simulink model "ArregloSeisPorSeis"
settings: Solver=ode23t  StartTime=0.0  StopTime=0.003  RelTol=1e-9  AbsTol=1e-9
values from neighbouring files (symbols this model uses):
  a11 = 300    [matlab1.mat]
  a12 = 200    [matlab1.mat]
  a13 = 100    [matlab1.mat]
  a14 = 100    [matlab1.mat]
  a15 = 100    [matlab1.mat]
  a16 = 100    [matlab1.mat]
  a21 = 200    [matlab1.mat]
  a22 = 100    [matlab1.mat]
  a23 = 100    [matlab1.mat]
  a24 = 1000    [matlab1.mat]
  a25 = 100    [matlab1.mat]
  a26 = 100    [matlab1.mat]
  a31 = 100    [matlab1.mat]
  a32 = 100    [matlab1.mat]
  a33 = 100    [matlab1.mat]
  a34 = 100    [matlab1.mat]
  a35 = 100    [matlab1.mat]
  a36 = 100    [matlab1.mat]
  a41 = 100    [matlab1.mat]
  a42 = 100    [matlab1.mat]
  a43 = 100    [matlab1.mat]
  a44 = 100    [matlab1.mat]
  a45 = 100    [matlab1.mat]
  a46 = 100    [matlab1.mat]
  a51 = 100    [matlab1.mat]
  a52 = 100    [matlab1.mat]
  a53 = 100    [matlab1.mat]
  a54 = 100    [matlab1.mat]
  a55 = 100    [matlab1.mat]
  a56 = 100    [matlab1.mat]
  a61 = 100    [matlab1.mat]
  a62 = 100    [matlab1.mat]
  a63 = 100    [matlab1.mat]
  a64 = 100    [matlab1.mat]
  a65 = 100    [matlab1.mat]
  a66 = 100    [matlab1.mat]
libraries: powerlib x154
(part 1 of 2)
settings Model: Creator=XUAN TRUONG  LastModifiedBy=David
settings SolverCC: AlgebraicLoopSolver=LineSearch  SolverResetMethod=Robust
settings DataIOCC: LimitDataPoints=on  SaveFormat=Array  SignalLoggingSaveFormat=ModelDataLogs  ReturnWorkspaceOutputs=off
settings OptimizationCC: ExpressionDepthLimit=2147483647  LifeSpan=inf  SimCompilerOptimization=Off
settings DebuggingCC: UnderspecifiedInitializationDetection=Classic  MergeDetectMultiDrivingBlocksExec=none  SolverPrmCheckMsg=warning  MultiTaskDSMMsg=warning  MultiTaskCondExecSysMsg=none  FcnCallInpInsideContextMsg=Enable All  StateNameClashWarn=warning  StrictBusMsg=None  SFUnexpectedBacktrackingDiag=warning  SFNoUnconditionalDefaultTransitionDiag=warning
settings HardwareCC: ProdBitPerPointer=32  ProdLargestAtomicFloat=None  ProdIntDivRoundTo=Undefined  ProdEndianess=Unspecified  ProdWordSize=32  ProdHWDeviceType=32-bit Generic
settings ModelReferenceCC: PropagateSignalLabelsOutOfModel=off
settings SFSimCC: SimUseLocalCustomCode=off
settings RTWCC: RTWUseLocalCustomCode=off  IncludeERTFirstTime=on  RTWCompilerOptimization=Off
settings GRTTargetCC: CodeReplacementLibrary=C89/C90 (ANSI)  GeneratePreprocessorConditionals=Disable all  CombineOutputUpdateFcns=off  CPPClassGenCompliant=off  GRTInterface=on

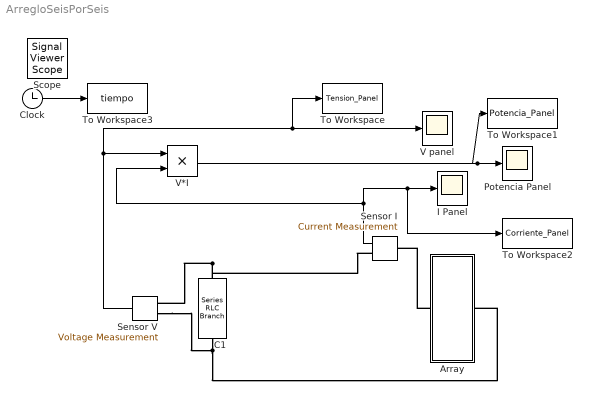
== system ArregloSeisPorSeis ==
  " C1" : powerlib/Elements/Series RLC Branch  LConnTagsString=__new0  RConnTagsString=__new0  BranchType=C  Resistance=5  Inductance=0.05  SetiL0=off  InitialCurrent=0  Capacitance=50e-6  Setx0=on  InitialVoltage=0  Measurements=Branch voltage and current
  Array : Subsystem
  Clock : Clock
  I Panel : Scope
      settings: YMin=0.00012  YMax=0.000137  SaveName=Ip  MaxDataPoints=150000
  Potencia Panel : Scope
      settings: TimeRange=0.003  YMin=0.01  YMax=0.0135  SaveName=P  MaxDataPoints=150000
  Sensor I : powerlib/Measurements/Current Measurement  PhasorSimulation=off  OutputType=Complex  PSBequivalent=0
  Sensor V : powerlib/Measurements/Voltage Measurement  PhasorSimulation=off  OutputType=Complex  PSBequivalent=0
  To Workspace : ToWorkspace  VariableName=Tension_Panel  SampleTime=-1
  To Workspace1 : ToWorkspace  VariableName=Potencia_Panel  SampleTime=-1
  To Workspace2 : ToWorkspace  VariableName=Corriente_Panel  SampleTime=-1
  To Workspace3 : ToWorkspace  VariableName=tiempo  SampleTime=-1
  V panel : Scope
      settings: YMin=130.2  YMax=130.9  SaveName=Vp  MaxDataPoints=150000
  V*I : Product  RndMeth=Zero
  Scope : SignalViewerScope  IOType=viewer  RefreshTime=0.035000
  wires:
  Sensor V/1 -> V*I/1, V panel/1, To Workspace/1
  Sensor I/1 -> V*I/2, I Panel/1, To Workspace2/1
  V*I/1 -> Potencia Panel/1, To Workspace1/1
  Clock/1 -> To Workspace3/1
  connections:
  " C1"/RConn1 -- Sensor V/LConn2 -- Array/RConn1
  " C1"/LConn1 -- Sensor I/RConn1 -- Sensor V/LConn1
  Array/LConn1 -- Sensor I/LConn1

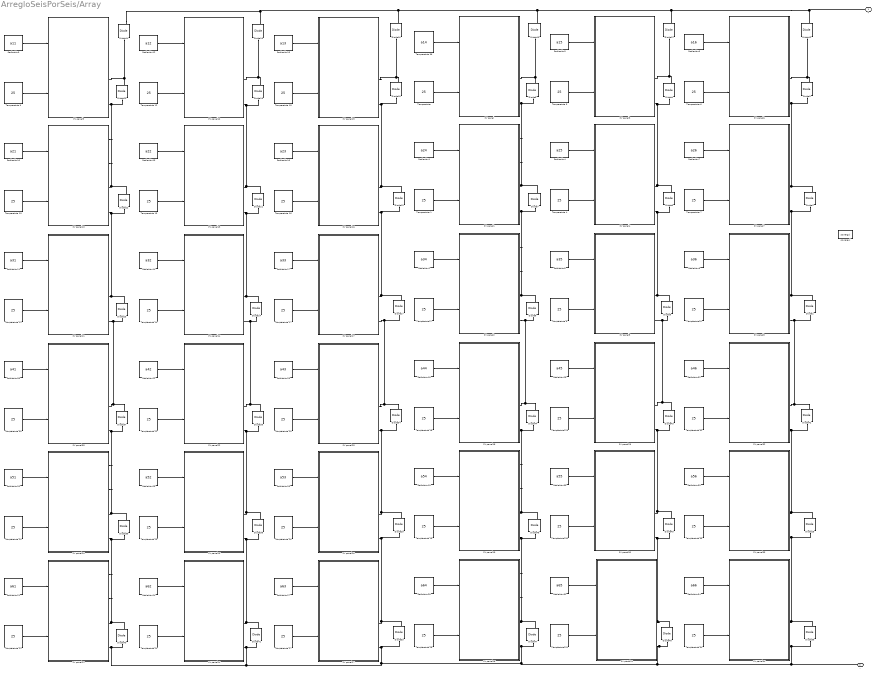
== system ArregloSeisPorSeis/Array ==
  Diode{1..25,29,33..48} (42 alike) : powerlib/Power Electronics/Diode  Ron=0.00001  Lon=0  Vf=0.3  IC=0  UseSnubber=off  Rs=1e10  Cs=1e-9  Measurements=on
  PV panel : Subsystem
      mask Display: image('C:\Users\Mauro\Dropbox\Fuente\Panel (2).jpg')
  PV panel1 : Subsystem
      mask Display: image('C:\Users\Mauro\Dropbox\Fuente\Panel (2).jpg')
  PV panel10 : Subsystem
      mask Display: image('C:\Users\Mauro\Dropbox\Fuente\Panel (2).jpg')
  PV panel11 : Subsystem
      mask Display: image('C:\Users\Mauro\Dropbox\Fuente\Panel (2).jpg')
  PV panel12 : Subsystem
      mask Display: image('C:\Users\Mauro\Dropbox\Fuente\Panel (2).jpg')
  PV panel13 : Subsystem
      mask Display: image('C:\Users\Mauro\Dropbox\Fuente\Panel (2).jpg')
  PV panel14 : Subsystem
      mask Display: image('C:\Users\Mauro\Dropbox\Fuente\Panel (2).jpg')
  PV panel15 : Subsystem
      mask Display: image('C:\Users\Mauro\Dropbox\Fuente\Panel (2).jpg')
  PV panel16 : Subsystem
      mask Display: image('C:\Users\Mauro\Dropbox\Fuente\Panel (2).jpg')
  PV panel17 : Subsystem
      mask Display: image('C:\Users\Mauro\Dropbox\Fuente\Panel (2).jpg')
  PV panel18 : Subsystem
      mask Display: image('C:\Users\Mauro\Dropbox\Fuente\Panel (2).jpg')
  PV panel19 : Subsystem
      mask Display: image('C:\Users\Mauro\Dropbox\Fuente\Panel (2).jpg')
  PV panel2 : Subsystem
      mask Display: image('C:\Users\Mauro\Dropbox\Fuente\Panel (2).jpg')
  PV panel20 : Subsystem
      mask Display: image('C:\Users\Mauro\Dropbox\Fuente\Panel (2).jpg')
  PV panel21 : Subsystem
      mask Display: image('C:\Users\Mauro\Dropbox\Fuente\Panel (2).jpg')
  PV panel22 : Subsystem
      mask Display: image('C:\Users\Mauro\Dropbox\Fuente\Panel (2).jpg')
  PV panel23 : Subsystem
      mask Display: image('C:\Users\Mauro\Dropbox\Fuente\Panel (2).jpg')
  PV panel24 : Subsystem
      mask Display: image('C:\Users\Mauro\Dropbox\Fuente\Panel (2).jpg')
  PV panel25 : Subsystem
      mask Display: image('C:\Users\Mauro\Dropbox\Fuente\Panel (2).jpg')
  PV panel26 : Subsystem
      mask Display: image('C:\Users\Mauro\Dropbox\Fuente\Panel (2).jpg')
  PV panel27 : Subsystem
      mask Display: image('C:\Users\Mauro\Dropbox\Fuente\Panel (2).jpg')
  PV panel28 : Subsystem
      mask Display: image('C:\Users\Mauro\Dropbox\Fuente\Panel (2).jpg')
  PV panel29 : Subsystem
      mask Display: image('C:\Users\Mauro\Dropbox\Fuente\Panel (2).jpg')
  PV panel3 : Subsystem
      mask Display: image('C:\Users\Mauro\Dropbox\Fuente\Panel (2).jpg')
  PV panel30 : Subsystem
      mask Display: image('C:\Users\Mauro\Dropbox\Fuente\Panel (2).jpg')
  PV panel31 : Subsystem
      mask Display: image('C:\Users\Mauro\Dropbox\Fuente\Panel (2).jpg')
  PV panel32 : Subsystem
      mask Display: image('C:\Users\Mauro\Dropbox\Fuente\Panel (2).jpg')
  PV panel33 : Subsystem
      mask Display: image('C:\Users\Mauro\Dropbox\Fuente\Panel (2).jpg')
  PV panel34 : Subsystem
      mask Display: image('C:\Users\Mauro\Dropbox\Fuente\Panel (2).jpg')
  PV panel35 : Subsystem
      mask Display: image('C:\Users\Mauro\Dropbox\Fuente\Panel (2).jpg')
  PV panel4 : Subsystem
      mask Display: image('C:\Users\Mauro\Dropbox\Fuente\Panel (2).jpg')
  PV panel5 : Subsystem
      mask Display: image('C:\Users\Mauro\Dropbox\Fuente\Panel (2).jpg')
  PV panel6 : Subsystem
      mask Display: image('C:\Users\Mauro\Dropbox\Fuente\Panel (2).jpg')
  PV panel7 : Subsystem
      mask Display: image('C:\Users\Mauro\Dropbox\Fuente\Panel (2).jpg')
  PV panel8 : Subsystem
      mask Display: image('C:\Users\Mauro\Dropbox\Fuente\Panel (2).jpg')
  PV panel9 : Subsystem
      mask Display: image('C:\Users\Mauro\Dropbox\Fuente\Panel (2).jpg')
  Radiación1 : Constant  Value=a24
      mask Display: image('C:\Users\Mauro\Dropbox\Fuente\Sol.jpg')
  Radiación10 : Constant  Value=a21
      mask Display: image('C:\Users\Mauro\Dropbox\Fuente\Sol.jpg')
  Radiación11 : Constant  Value=a31
      mask Display: image('C:\Users\Mauro\Dropbox\Fuente\Sol.jpg')
  Radiación12 : Constant  Value=a12
      mask Display: image('C:\Users\Mauro\Dropbox\Fuente\Sol.jpg')
  Radiación13 : Constant  Value=a22
      mask Display: image('C:\Users\Mauro\Dropbox\Fuente\Sol.jpg')
  Radiación14 : Constant  Value=a32
      mask Display: image('C:\Users\Mauro\Dropbox\Fuente\Sol.jpg')
  Radiación15 : Constant  Value=a13
      mask Display: image('C:\Users\Mauro\Dropbox\Fuente\Sol.jpg')
  Radiación16 : Constant  Value=a23
      mask Display: image('C:\Users\Mauro\Dropbox\Fuente\Sol.jpg')
  Radiación17 : Constant  Value=a33
      mask Display: image('C:\Users\Mauro\Dropbox\Fuente\Sol.jpg')
  Radiación18 : Constant  Value=a44
      mask Display: image('C:\Users\Mauro\Dropbox\Fuente\Sol.jpg')
  Radiación19 : Constant  Value=a54
      mask Display: image('C:\Users\Mauro\Dropbox\Fuente\Sol.jpg')
  Radiación2 : Constant  Value=a34
      mask Display: image('C:\Users\Mauro\Dropbox\Fuente\Sol.jpg')
  Radiación20 : Constant  Value=a51
      mask Display: image('C:\Users\Mauro\Dropbox\Fuente\Sol.jpg')
  Radiación21 : Constant  Value=a61
      mask Display: image('C:\Users\Mauro\Dropbox\Fuente\Sol.jpg')
  Radiación22 : Constant  Value=a42
      mask Display: image('C:\Users\Mauro\Dropbox\Fuente\Sol.jpg')
  Radiación23 : Constant  Value=a52
      mask Display: image('C:\Users\Mauro\Dropbox\Fuente\Sol.jpg')
  Radiación24 : Constant  Value=a62
      mask Display: image('C:\Users\Mauro\Dropbox\Fuente\Sol.jpg')
  Radiación25 : Constant  Value=a43
      mask Display: image('C:\Users\Mauro\Dropbox\Fuente\Sol.jpg')
  Radiación26 : Constant  Value=a53
      mask Display: image('C:\Users\Mauro\Dropbox\Fuente\Sol.jpg')
  Radiación27 : Constant  Value=a63
      mask Display: image('C:\Users\Mauro\Dropbox\Fuente\Sol.jpg')
  Radiación28 : Constant  Value=a64
      mask Display: image('C:\Users\Mauro\Dropbox\Fuente\Sol.jpg')
  Radiación29 : Constant  Value=a45
      mask Display: image('C:\Users\Mauro\Dropbox\Fuente\Sol.jpg')
  Radiación3 : Constant  Value=a15
      mask Display: image('C:\Users\Mauro\Dropbox\Fuente\Sol.jpg')
  Radiación30 : Constant  Value=a55
      mask Display: image('C:\Users\Mauro\Dropbox\Fuente\Sol.jpg')
  Radiación31 : Constant  Value=a65
      mask Display: image('C:\Users\Mauro\Dropbox\Fuente\Sol.jpg')
  Radiación32 : Constant  Value=a46
      mask Display: image('C:\Users\Mauro\Dropbox\Fuente\Sol.jpg')
  Radiación33 : Constant  Value=a56
      mask Display: image('C:\Users\Mauro\Dropbox\Fuente\Sol.jpg')
  Radiación34 : Constant  Value=a66
      mask Display: image('C:\Users\Mauro\Dropbox\Fuente\Sol.jpg')
  Radiación35 : Constant  Value=a41
      mask Display: image('C:\Users\Mauro\Dropbox\Fuente\Sol.jpg')
  Radiación4 : Constant  Value=a25
      mask Display: image('C:\Users\Mauro\Dropbox\Fuente\Sol.jpg')
  Radiación5 : Constant  Value=a35
      mask Display: image('C:\Users\Mauro\Dropbox\Fuente\Sol.jpg')
  Radiación6 : Constant  Value=a16
      mask Display: image('C:\Users\Mauro\Dropbox\Fuente\Sol.jpg')
  Radiación7 : Constant  Value=a26
      mask Display: image('C:\Users\Mauro\Dropbox\Fuente\Sol.jpg')
  Radiación8 : Constant  Value=a36
      mask Display: image('C:\Users\Mauro\Dropbox\Fuente\Sol.jpg')
  Radiación9 : Constant  Value=a11
      mask Display: image('C:\Users\Mauro\Dropbox\Fuente\Sol.jpg')
  Temperatuta {,1..35} (36 alike) : Constant  Value=25
      mask Display: image('C:\Users\Mauro\Dropbox\Fuente\Termometro.jpg')
  Temperatuta 36 : Constant  Value=a14
      mask Display: image('C:\Users\Mauro\Dropbox\Fuente\Termometro.jpg')
  powergui : powerlib/powergui  Priority=1  SimulationMode=Discrete  SolverType=Tustin  SampleTime=5e-6  frequency=60  SPID=off  DisableSnubberDevices=off  DisableRonSwitches=off  DisableVfSwitches=off  SwTol=0  Interpol=off  DisplayEquations=off  FunctionMessages=off  frequencyindice=0  Pbase=100e6  ErrMax=1e-4  Iterations=50  UnitsV=kV  UnitsW=MW  echomessages=off  HookPort=off  EnableUseOfTLC=off  x0status=blocks  RestoreLinks=warning  ResistiveCurrentMeasurement=off  Frange=[0:2:500]  Ylog=off  Xlog=on  ShowGrid=off  save=off  variable=ZData  ZoomFFT=off  StartTime=0.0  cycles=1  DisplayStyle=1  fundamental=60  FreqAxis=off  MaxFrequency=1000  frequencyindicesteady=1  RmsSteady=1  display=off  Ts=0  methode=off
  + : PMIOPort  Tag=PMCPort  Port=1  Side=Left
  - : PMIOPort  Tag=PMCPort  Port=2  Side=Right
  wires:
  Radiación2/1 -> PV panel2/1(Radiación)
  Temperatuta 2/1 -> PV panel2/2(Temperatura)
  Radiación3/1 -> PV panel3/1(Radiación)
  Temperatuta 3/1 -> PV panel3/2(Temperatura)
  Radiación4/1 -> PV panel4/1(Radiación)
  Temperatuta 4/1 -> PV panel4/2(Temperatura)
  Radiación5/1 -> PV panel5/1(Radiación)
  Temperatuta 5/1 -> PV panel5/2(Temperatura)
  PV panel1/1(Ipv) -> ?
  PV panel1/2(Vpv) -> ?
  Radiación6/1 -> PV panel6/1(Radiación)
  Temperatuta 6/1 -> PV panel6/2(Temperatura)
  Radiación7/1 -> PV panel7/1(Radiación)
  Temperatuta 7/1 -> PV panel7/2(Temperatura)
  Radiación8/1 -> PV panel8/1(Radiación)
  Temperatuta 8/1 -> PV panel8/2(Temperatura)
  Temperatuta 36/1 -> PV panel/1(Radiación)
  "Temperatuta "/1 -> PV panel/2(Temperatura)
  Radiación1/1 -> PV panel1/1(Radiación)
  Temperatuta 1/1 -> PV panel1/2(Temperatura)
  PV panel2/2(Vpv) -> ?
  PV panel2/1(Ipv) -> ?
  Radiación11/1 -> PV panel11/1(Radiación)
  Temperatuta 11/1 -> PV panel11/2(Temperatura)
  Radiación12/1 -> PV panel12/1(Radiación)
  Temperatuta 12/1 -> PV panel12/2(Temperatura)
  Radiación13/1 -> PV panel13/1(Radiación)
  Temperatuta 13/1 -> PV panel13/2(Temperatura)
  Radiación14/1 -> PV panel14/1(Radiación)
  Temperatuta 14/1 -> PV panel14/2(Temperatura)
  PV panel10/1(Ipv) -> ?
  PV panel10/2(Vpv) -> ?
  Radiación15/1 -> PV panel15/1(Radiación)
  Temperatuta 15/1 -> PV panel15/2(Temperatura)
  Radiación16/1 -> PV panel16/1(Radiación)
  Temperatuta 16/1 -> PV panel16/2(Temperatura)
  Radiación17/1 -> PV panel17/1(Radiación)
  Temperatuta 17/1 -> PV panel17/2(Temperatura)
  Radiación9/1 -> PV panel9/1(Radiación)
  Temperatuta 9/1 -> PV panel9/2(Temperatura)
  Radiación10/1 -> PV panel10/1(Radiación)
  Temperatuta 10/1 -> PV panel10/2(Temperatura)
  Radiación28/1 -> PV panel28/1(Radiación)
  Temperatuta 28/1 -> PV panel28/2(Temperatura)
  Radiación29/1 -> PV panel29/1(Radiación)
  Temperatuta 29/1 -> PV panel29/2(Temperatura)
  Radiación30/1 -> PV panel30/1(Radiación)
  Temperatuta 30/1 -> PV panel30/2(Temperatura)
  Radiación31/1 -> PV panel31/1(Radiación)
  Temperatuta 31/1 -> PV panel31/2(Temperatura)
  PV panel19/1(Ipv) -> ?
  PV panel19/2(Vpv) -> ?
  Radiación32/1 -> PV panel32/1(Radiación)
  Temperatuta 32/1 -> PV panel32/2(Temperatura)
  Radiación33/1 -> PV panel33/1(Radiación)
  Temperatuta 33/1 -> PV panel33/2(Temperatura)
  Radiación34/1 -> PV panel34/1(Radiación)
  Temperatuta 34/1 -> PV panel34/2(Temperatura)
  Radiación18/1 -> PV panel18/1(Radiación)
  Temperatuta 18/1 -> PV panel18/2(Temperatura)
  Radiación19/1 -> PV panel19/1(Radiación)
  Temperatuta 19/1 -> PV panel19/2(Temperatura)
  PV panel28/2(Vpv) -> ?
  PV panel28/1(Ipv) -> ?
  Radiación21/1 -> PV panel21/1(Radiación)
  Temperatuta 21/1 -> PV panel21/2(Temperatura)
  Radiación22/1 -> PV panel22/1(Radiación)
  Temperatuta 22/1 -> PV panel22/2(Temperatura)
  Radiación23/1 -> PV panel23/1(Radiación)
  Temperatuta 23/1 -> PV panel23/2(Temperatura)
  Radiación24/1 -> PV panel24/1(Radiación)
  Temperatuta 24/1 -> PV panel24/2(Temperatura)
  PV panel20/1(Ipv) -> ?
  PV panel20/2(Vpv) -> ?
  Radiación25/1 -> PV panel25/1(Radiación)
  Temperatuta 25/1 -> PV panel25/2(Temperatura)
  Radiación26/1 -> PV panel26/1(Radiación)
  Temperatuta 26/1 -> PV panel26/2(Temperatura)
  Radiación27/1 -> PV panel27/1(Radiación)
  Temperatuta 27/1 -> PV panel27/2(Temperatura)
  Radiación35/1 -> PV panel35/1(Radiación)
  Temperatuta 35/1 -> PV panel35/2(Temperatura)
  Radiación20/1 -> PV panel20/1(Radiación)
  Temperatuta 20/1 -> PV panel20/2(Temperatura)
  PV panel21/2(Vpv) -> ?
  PV panel21/1(Ipv) -> ?
  connections:
  PV panel/RConn2 -- Diode5/LConn1 -- Diode7/RConn1 -- PV panel1/RConn1
  PV panel4/RConn1 -- Diode6/RConn1 -- Diode4/LConn1 -- PV panel3/RConn2
  PV panel7/RConn1 -- Diode1/RConn1 -- Diode3/LConn1 -- PV panel6/RConn2
  PV panel5/RConn1 -- Diode9/RConn1 -- Diode6/LConn1 -- PV panel4/RConn2
  Diode14/RConn1 -- Diode10/RConn1 -- +/RConn1 -- Diode12/RConn1 -- Diode11/RConn1 -- Diode16/RConn1 -- Diode15/RConn1
  PV panel2/RConn1 -- Diode8/RConn1 -- Diode7/LConn1 -- PV panel1/RConn2
  PV panel8/RConn1 -- Diode2/RConn1 -- Diode1/LConn1 -- PV panel7/RConn2
  PV panel18/RConn1 -- Diode44/RConn1 -- Diode8/LConn1 -- PV panel2/RConn2
  PV panel/RConn1 -- Diode5/RConn1 -- Diode10/LConn1
  Diode4/RConn1 -- Diode11/LConn1 -- PV panel3/RConn1
  PV panel6/RConn1 -- Diode3/RConn1 -- Diode12/LConn1
  PV panel9/RConn2 -- Diode20/LConn1 -- Diode22/RConn1 -- PV panel10/RConn1
  PV panel12/RConn2 -- Diode21/RConn1 -- PV panel13/RConn1 -- Diode19/LConn1
  PV panel16/RConn1 -- Diode13/RConn1 -- Diode18/LConn1 -- PV panel15/RConn2
  PV panel13/RConn2 -- Diode24/RConn1 -- PV panel14/RConn1 -- Diode21/LConn1
  PV panel10/RConn2 -- Diode23/RConn1 -- PV panel11/RConn1 -- Diode22/LConn1
  PV panel16/RConn2 -- Diode13/LConn1 -- Diode17/RConn1 -- PV panel17/RConn1
  PV panel9/RConn1 -- Diode20/RConn1 -- Diode14/LConn1
  Diode19/RConn1 -- Diode15/LConn1 -- PV panel12/RConn1
  PV panel15/RConn1 -- Diode18/RConn1 -- Diode16/LConn1
  PV panel18/RConn2 -- Diode44/LConn1 -- Diode46/RConn1 -- PV panel19/RConn1
  PV panel29/RConn2 -- Diode45/RConn1 -- PV panel30/RConn1 -- Diode43/LConn1
  PV panel33/RConn1 -- Diode25/RConn1 -- Diode42/LConn1 -- PV panel32/RConn2
  PV panel30/RConn2 -- Diode48/RConn1 -- PV panel31/RConn1 -- Diode45/LConn1
  PV panel19/RConn2 -- Diode47/RConn1 -- PV panel28/RConn1 -- Diode46/LConn1
  PV panel33/RConn2 -- Diode36/RConn1 -- PV panel34/RConn1 -- Diode25/LConn1
  PV panel27/RConn2 -- Diode33/LConn1 -- Diode36/LConn1 -- PV panel34/RConn2 -- -/RConn1 -- Diode48/LConn1 -- PV panel31/RConn2 -- Diode47/LConn1 -- PV panel28/RConn2 -- Diode40/LConn1 -- PV panel21/RConn2 -- Diode41/LConn1 -- PV panel24/RConn2
  PV panel35/RConn2 -- Diode37/LConn1 -- Diode39/RConn1 -- PV panel20/RConn1
  PV panel22/RConn2 -- Diode35/LConn1 -- Diode38/RConn1 -- PV panel23/RConn1
  PV panel26/RConn1 -- Diode29/RConn1 -- Diode34/LConn1 -- PV panel25/RConn2
  PV panel23/RConn2 -- Diode38/LConn1 -- Diode41/RConn1 -- PV panel24/RConn1
  PV panel20/RConn2 -- Diode39/LConn1 -- Diode40/RConn1 -- PV panel21/RConn1
  PV panel26/RConn2 -- Diode29/LConn1 -- Diode33/RConn1 -- PV panel27/RConn1
  PV panel32/RConn1 -- Diode42/RConn1 -- Diode2/LConn1 -- PV panel8/RConn2
  Diode43/RConn1 -- PV panel5/RConn2 -- Diode9/LConn1 -- PV panel29/RConn1
  Diode35/RConn1 -- PV panel14/RConn2 -- Diode24/LConn1 -- PV panel22/RConn1
  PV panel25/RConn1 -- Diode34/RConn1 -- Diode17/LConn1 -- PV panel17/RConn2
  PV panel35/RConn1 -- Diode23/LConn1 -- PV panel11/RConn2 -- Diode37/RConn1

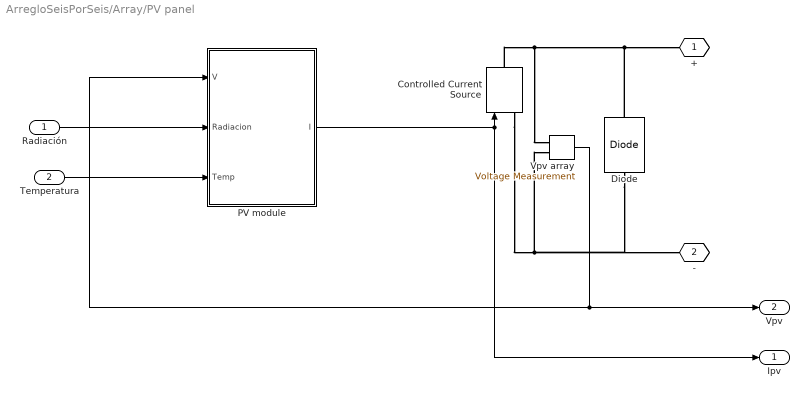
== system ArregloSeisPorSeis/Array/PV panel ==
  Radiación : Inport
  Temperatura : Inport  Port=2
  Controlled Current Source : powerlib/Electrical Sources/Controlled Current Source  Initialize=on  Source_Type=AC  Amplitude=0  Phase=0  Frequency=0  Measurements=None
  Diode : powerlib/Power Electronics/Diode  Ron=0.001  Lon=0  Vf=0  IC=0  UseSnubber=off  Rs=500  Cs=250e-9  Measurements=off
  PV module : MATLAB Function  TreatAsAtomicUnit=on
  Vpv array : powerlib/Measurements/Voltage Measurement  PhasorSimulation=off  OutputType=Complex  PSBequivalent=0
  + : PMIOPort  Tag=PMCPort  Port=1  Side=Right
  - : PMIOPort  Tag=PMCPort  Port=2  Side=Right
  Ipv : Outport
  Vpv : Outport  Port=2
  wires:
  Radiación/1 -> PV module/2(Radiacion)
  Temperatura/1 -> PV module/3(Temp)
  PV module/1(I) -> Controlled Current Source/1, Ipv/1
  Vpv array/1 -> PV module/1(V), Vpv/1
  connections:
  Controlled Current Source/LConn1 -- Diode/LConn1 -- -/RConn1 -- Vpv array/LConn2
  Controlled Current Source/RConn1 -- Diode/RConn1 -- +/RConn1 -- Vpv array/LConn1

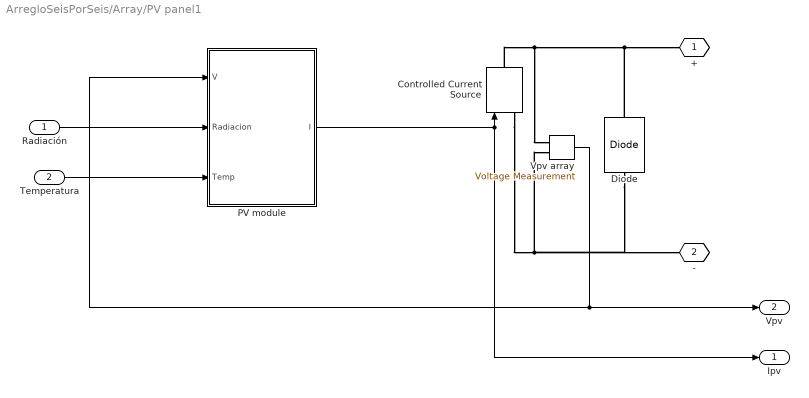
== system ArregloSeisPorSeis/Array/PV panel1 ==
  Radiación : Inport
  Temperatura : Inport  Port=2
  Controlled Current Source : powerlib/Electrical Sources/Controlled Current Source  Initialize=on  Source_Type=AC  Amplitude=0  Phase=0  Frequency=0  Measurements=None
  Diode : powerlib/Power Electronics/Diode  Ron=0.001  Lon=0  Vf=0  IC=0  UseSnubber=off  Rs=500  Cs=250e-9  Measurements=off
  PV module : MATLAB Function  TreatAsAtomicUnit=on
  Vpv array : powerlib/Measurements/Voltage Measurement  PhasorSimulation=off  OutputType=Complex  PSBequivalent=0
  + : PMIOPort  Tag=PMCPort  Port=1  Side=Right
  - : PMIOPort  Tag=PMCPort  Port=2  Side=Right
  Ipv : Outport
  Vpv : Outport  Port=2
  wires:
  Radiación/1 -> PV module/2(Radiacion)
  Temperatura/1 -> PV module/3(Temp)
  PV module/1(I) -> Controlled Current Source/1, Ipv/1
  Vpv array/1 -> PV module/1(V), Vpv/1
  connections:
  Controlled Current Source/LConn1 -- Diode/LConn1 -- -/RConn1 -- Vpv array/LConn2
  Controlled Current Source/RConn1 -- Diode/RConn1 -- +/RConn1 -- Vpv array/LConn1

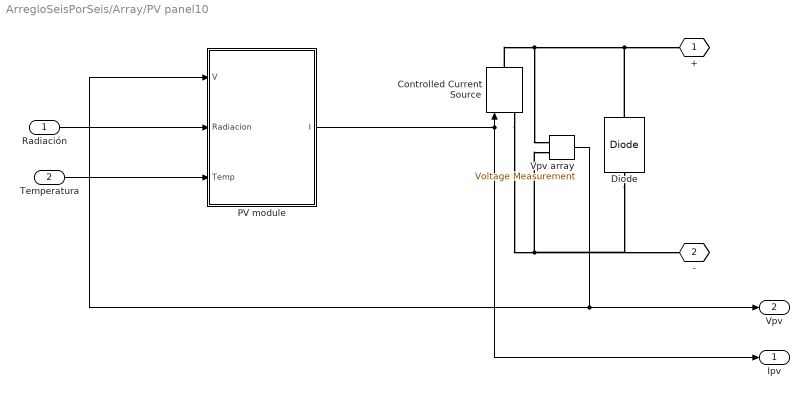
== system ArregloSeisPorSeis/Array/PV panel10 ==
  Radiación : Inport
  Temperatura : Inport  Port=2
  Controlled Current Source : powerlib/Electrical Sources/Controlled Current Source  Initialize=on  Source_Type=AC  Amplitude=0  Phase=0  Frequency=0  Measurements=None
  Diode : powerlib/Power Electronics/Diode  Ron=0.001  Lon=0  Vf=0  IC=0  UseSnubber=off  Rs=500  Cs=250e-9  Measurements=off
  PV module : MATLAB Function  TreatAsAtomicUnit=on
  Vpv array : powerlib/Measurements/Voltage Measurement  PhasorSimulation=off  OutputType=Complex  PSBequivalent=0
  + : PMIOPort  Tag=PMCPort  Port=1  Side=Right
  - : PMIOPort  Tag=PMCPort  Port=2  Side=Right
  Ipv : Outport
  Vpv : Outport  Port=2
  wires:
  Radiación/1 -> PV module/2(Radiacion)
  Temperatura/1 -> PV module/3(Temp)
  PV module/1(I) -> Controlled Current Source/1, Ipv/1
  Vpv array/1 -> PV module/1(V), Vpv/1
  connections:
  Controlled Current Source/LConn1 -- Diode/LConn1 -- -/RConn1 -- Vpv array/LConn2
  Controlled Current Source/RConn1 -- Diode/RConn1 -- +/RConn1 -- Vpv array/LConn1

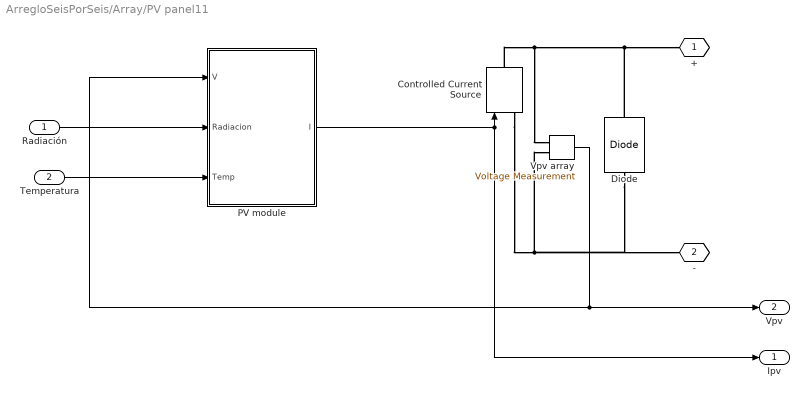
== system ArregloSeisPorSeis/Array/PV panel11 ==
  Radiación : Inport
  Temperatura : Inport  Port=2
  Controlled Current Source : powerlib/Electrical Sources/Controlled Current Source  Initialize=on  Source_Type=AC  Amplitude=0  Phase=0  Frequency=0  Measurements=None
  Diode : powerlib/Power Electronics/Diode  Ron=0.001  Lon=0  Vf=0  IC=0  UseSnubber=off  Rs=500  Cs=250e-9  Measurements=off
  PV module : MATLAB Function  TreatAsAtomicUnit=on
  Vpv array : powerlib/Measurements/Voltage Measurement  PhasorSimulation=off  OutputType=Complex  PSBequivalent=0
  + : PMIOPort  Tag=PMCPort  Port=1  Side=Right
  - : PMIOPort  Tag=PMCPort  Port=2  Side=Right
  Ipv : Outport
  Vpv : Outport  Port=2
  wires:
  Radiación/1 -> PV module/2(Radiacion)
  Temperatura/1 -> PV module/3(Temp)
  PV module/1(I) -> Controlled Current Source/1, Ipv/1
  Vpv array/1 -> PV module/1(V), Vpv/1
  connections:
  Controlled Current Source/LConn1 -- Diode/LConn1 -- -/RConn1 -- Vpv array/LConn2
  Controlled Current Source/RConn1 -- Diode/RConn1 -- +/RConn1 -- Vpv array/LConn1

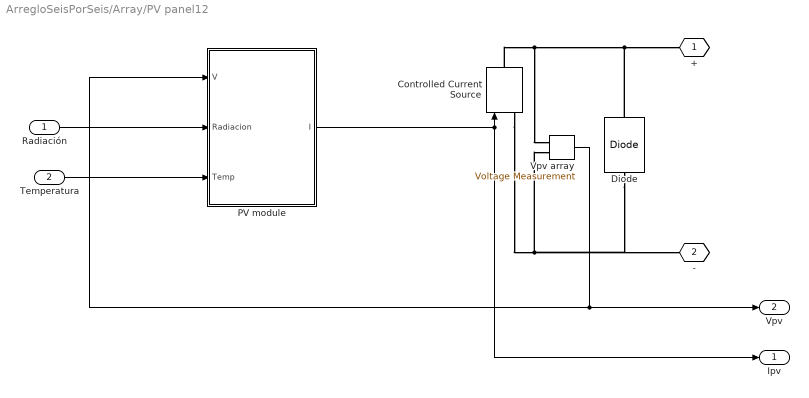
== system ArregloSeisPorSeis/Array/PV panel12 ==
  Radiación : Inport
  Temperatura : Inport  Port=2
  Controlled Current Source : powerlib/Electrical Sources/Controlled Current Source  Initialize=on  Source_Type=AC  Amplitude=0  Phase=0  Frequency=0  Measurements=None
  Diode : powerlib/Power Electronics/Diode  Ron=0.001  Lon=0  Vf=0  IC=0  UseSnubber=off  Rs=500  Cs=250e-9  Measurements=off
  PV module : MATLAB Function  TreatAsAtomicUnit=on
  Vpv array : powerlib/Measurements/Voltage Measurement  PhasorSimulation=off  OutputType=Complex  PSBequivalent=0
  + : PMIOPort  Tag=PMCPort  Port=1  Side=Right
  - : PMIOPort  Tag=PMCPort  Port=2  Side=Right
  Ipv : Outport
  Vpv : Outport  Port=2
  wires:
  Radiación/1 -> PV module/2(Radiacion)
  Temperatura/1 -> PV module/3(Temp)
  PV module/1(I) -> Controlled Current Source/1, Ipv/1
  Vpv array/1 -> PV module/1(V), Vpv/1
  connections:
  Controlled Current Source/LConn1 -- Diode/LConn1 -- -/RConn1 -- Vpv array/LConn2
  Controlled Current Source/RConn1 -- Diode/RConn1 -- +/RConn1 -- Vpv array/LConn1

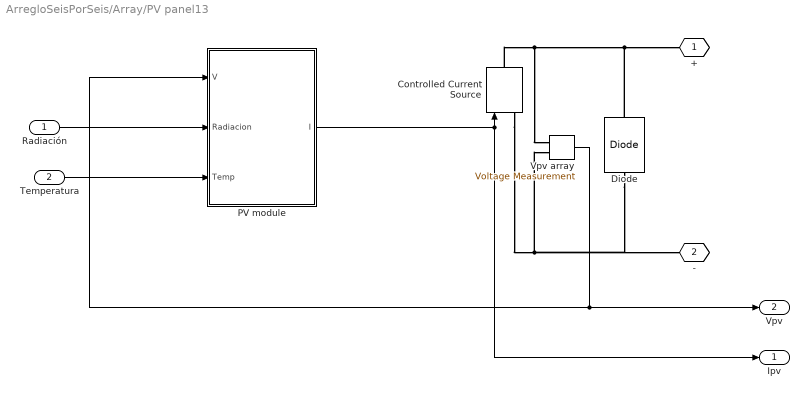
== system ArregloSeisPorSeis/Array/PV panel13 ==
  Radiación : Inport
  Temperatura : Inport  Port=2
  Controlled Current Source : powerlib/Electrical Sources/Controlled Current Source  Initialize=on  Source_Type=AC  Amplitude=0  Phase=0  Frequency=0  Measurements=None
  Diode : powerlib/Power Electronics/Diode  Ron=0.001  Lon=0  Vf=0  IC=0  UseSnubber=off  Rs=500  Cs=250e-9  Measurements=off
  PV module : MATLAB Function  TreatAsAtomicUnit=on
  Vpv array : powerlib/Measurements/Voltage Measurement  PhasorSimulation=off  OutputType=Complex  PSBequivalent=0
  + : PMIOPort  Tag=PMCPort  Port=1  Side=Right
  - : PMIOPort  Tag=PMCPort  Port=2  Side=Right
  Ipv : Outport
  Vpv : Outport  Port=2
  wires:
  Radiación/1 -> PV module/2(Radiacion)
  Temperatura/1 -> PV module/3(Temp)
  PV module/1(I) -> Controlled Current Source/1, Ipv/1
  Vpv array/1 -> PV module/1(V), Vpv/1
  connections:
  Controlled Current Source/LConn1 -- Diode/LConn1 -- -/RConn1 -- Vpv array/LConn2
  Controlled Current Source/RConn1 -- Diode/RConn1 -- +/RConn1 -- Vpv array/LConn1

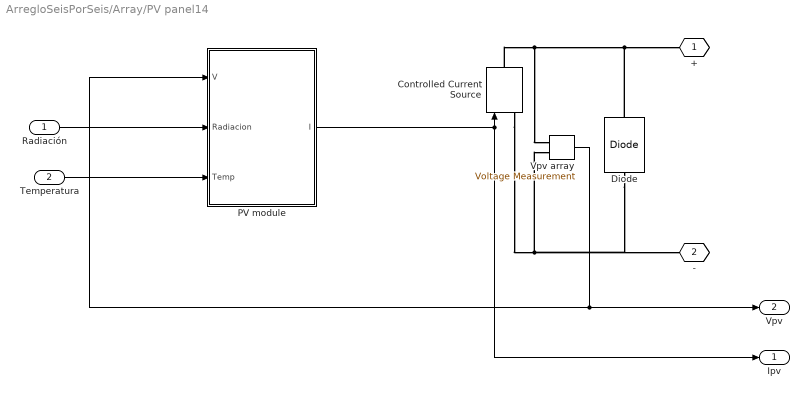
== system ArregloSeisPorSeis/Array/PV panel14 ==
  Radiación : Inport
  Temperatura : Inport  Port=2
  Controlled Current Source : powerlib/Electrical Sources/Controlled Current Source  Initialize=on  Source_Type=AC  Amplitude=0  Phase=0  Frequency=0  Measurements=None
  Diode : powerlib/Power Electronics/Diode  Ron=0.001  Lon=0  Vf=0  IC=0  UseSnubber=off  Rs=500  Cs=250e-9  Measurements=off
  PV module : MATLAB Function  TreatAsAtomicUnit=on
  Vpv array : powerlib/Measurements/Voltage Measurement  PhasorSimulation=off  OutputType=Complex  PSBequivalent=0
  + : PMIOPort  Tag=PMCPort  Port=1  Side=Right
  - : PMIOPort  Tag=PMCPort  Port=2  Side=Right
  Ipv : Outport
  Vpv : Outport  Port=2
  wires:
  Radiación/1 -> PV module/2(Radiacion)
  Temperatura/1 -> PV module/3(Temp)
  PV module/1(I) -> Controlled Current Source/1, Ipv/1
  Vpv array/1 -> PV module/1(V), Vpv/1
  connections:
  Controlled Current Source/LConn1 -- Diode/LConn1 -- -/RConn1 -- Vpv array/LConn2
  Controlled Current Source/RConn1 -- Diode/RConn1 -- +/RConn1 -- Vpv array/LConn1

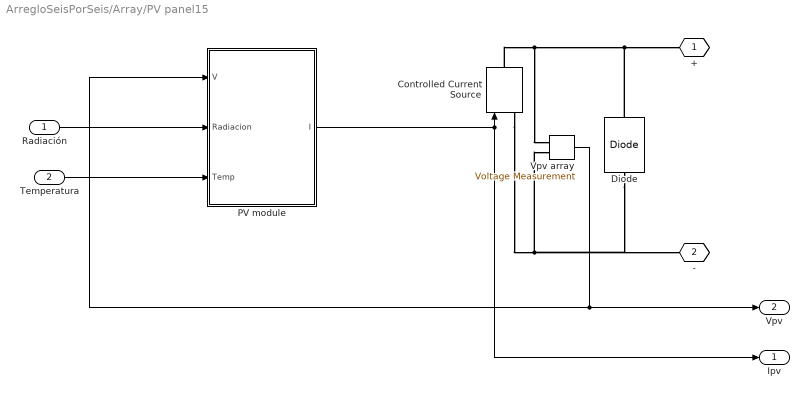
== system ArregloSeisPorSeis/Array/PV panel15 ==
  Radiación : Inport
  Temperatura : Inport  Port=2
  Controlled Current Source : powerlib/Electrical Sources/Controlled Current Source  Initialize=on  Source_Type=AC  Amplitude=0  Phase=0  Frequency=0  Measurements=None
  Diode : powerlib/Power Electronics/Diode  Ron=0.001  Lon=0  Vf=0  IC=0  UseSnubber=off  Rs=500  Cs=250e-9  Measurements=off
  PV module : MATLAB Function  TreatAsAtomicUnit=on
  Vpv array : powerlib/Measurements/Voltage Measurement  PhasorSimulation=off  OutputType=Complex  PSBequivalent=0
  + : PMIOPort  Tag=PMCPort  Port=1  Side=Right
  - : PMIOPort  Tag=PMCPort  Port=2  Side=Right
  Ipv : Outport
  Vpv : Outport  Port=2
  wires:
  Radiación/1 -> PV module/2(Radiacion)
  Temperatura/1 -> PV module/3(Temp)
  PV module/1(I) -> Controlled Current Source/1, Ipv/1
  Vpv array/1 -> PV module/1(V), Vpv/1
  connections:
  Controlled Current Source/LConn1 -- Diode/LConn1 -- -/RConn1 -- Vpv array/LConn2
  Controlled Current Source/RConn1 -- Diode/RConn1 -- +/RConn1 -- Vpv array/LConn1

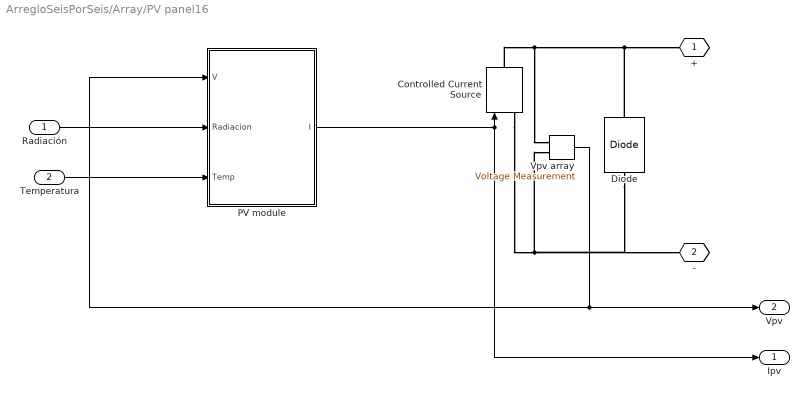
== system ArregloSeisPorSeis/Array/PV panel16 ==
  Radiación : Inport
  Temperatura : Inport  Port=2
  Controlled Current Source : powerlib/Electrical Sources/Controlled Current Source  Initialize=on  Source_Type=AC  Amplitude=0  Phase=0  Frequency=0  Measurements=None
  Diode : powerlib/Power Electronics/Diode  Ron=0.001  Lon=0  Vf=0  IC=0  UseSnubber=off  Rs=500  Cs=250e-9  Measurements=off
  PV module : MATLAB Function  TreatAsAtomicUnit=on
  Vpv array : powerlib/Measurements/Voltage Measurement  PhasorSimulation=off  OutputType=Complex  PSBequivalent=0
  + : PMIOPort  Tag=PMCPort  Port=1  Side=Right
  - : PMIOPort  Tag=PMCPort  Port=2  Side=Right
  Ipv : Outport
  Vpv : Outport  Port=2
  wires:
  Radiación/1 -> PV module/2(Radiacion)
  Temperatura/1 -> PV module/3(Temp)
  PV module/1(I) -> Controlled Current Source/1, Ipv/1
  Vpv array/1 -> PV module/1(V), Vpv/1
  connections:
  Controlled Current Source/LConn1 -- Diode/LConn1 -- -/RConn1 -- Vpv array/LConn2
  Controlled Current Source/RConn1 -- Diode/RConn1 -- +/RConn1 -- Vpv array/LConn1

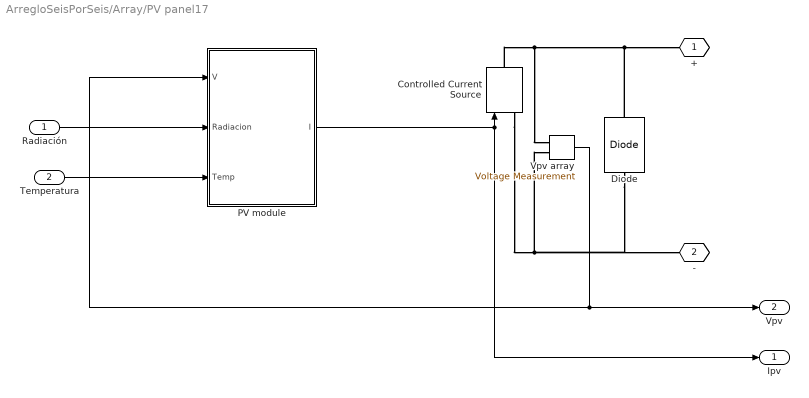
== system ArregloSeisPorSeis/Array/PV panel17 ==
  Radiación : Inport
  Temperatura : Inport  Port=2
  Controlled Current Source : powerlib/Electrical Sources/Controlled Current Source  Initialize=on  Source_Type=AC  Amplitude=0  Phase=0  Frequency=0  Measurements=None
  Diode : powerlib/Power Electronics/Diode  Ron=0.001  Lon=0  Vf=0  IC=0  UseSnubber=off  Rs=500  Cs=250e-9  Measurements=off
  PV module : MATLAB Function  TreatAsAtomicUnit=on
  Vpv array : powerlib/Measurements/Voltage Measurement  PhasorSimulation=off  OutputType=Complex  PSBequivalent=0
  + : PMIOPort  Tag=PMCPort  Port=1  Side=Right
  - : PMIOPort  Tag=PMCPort  Port=2  Side=Right
  Ipv : Outport
  Vpv : Outport  Port=2
  wires:
  Radiación/1 -> PV module/2(Radiacion)
  Temperatura/1 -> PV module/3(Temp)
  PV module/1(I) -> Controlled Current Source/1, Ipv/1
  Vpv array/1 -> PV module/1(V), Vpv/1
  connections:
  Controlled Current Source/LConn1 -- Diode/LConn1 -- -/RConn1 -- Vpv array/LConn2
  Controlled Current Source/RConn1 -- Diode/RConn1 -- +/RConn1 -- Vpv array/LConn1

== system ArregloSeisPorSeis/Array/PV panel18 ==
  Radiación : Inport
  Temperatura : Inport  Port=2
  Controlled Current Source : powerlib/Electrical Sources/Controlled Current Source  Initialize=on  Source_Type=AC  Amplitude=0  Phase=0  Frequency=0  Measurements=None
  Diode : powerlib/Power Electronics/Diode  Ron=0.001  Lon=0  Vf=0  IC=0  UseSnubber=off  Rs=500  Cs=250e-9  Measurements=off
  PV module : MATLAB Function  TreatAsAtomicUnit=on
  Vpv array : powerlib/Measurements/Voltage Measurement  PhasorSimulation=off  OutputType=Complex  PSBequivalent=0
  + : PMIOPort  Tag=PMCPort  Port=1  Side=Right
  - : PMIOPort  Tag=PMCPort  Port=2  Side=Right
  Ipv : Outport
  Vpv : Outport  Port=2
  wires:
  Radiación/1 -> PV module/2(Radiacion)
  Temperatura/1 -> PV module/3(Temp)
  PV module/1(I) -> Controlled Current Source/1, Ipv/1
  Vpv array/1 -> PV module/1(V), Vpv/1
  connections:
  Controlled Current Source/LConn1 -- Diode/LConn1 -- -/RConn1 -- Vpv array/LConn2
  Controlled Current Source/RConn1 -- Diode/RConn1 -- +/RConn1 -- Vpv array/LConn1

== system ArregloSeisPorSeis/Array/PV panel19 ==
  Radiación : Inport
  Temperatura : Inport  Port=2
  Controlled Current Source : powerlib/Electrical Sources/Controlled Current Source  Initialize=on  Source_Type=AC  Amplitude=0  Phase=0  Frequency=0  Measurements=None
  Diode : powerlib/Power Electronics/Diode  Ron=0.001  Lon=0  Vf=0  IC=0  UseSnubber=off  Rs=500  Cs=250e-9  Measurements=off
  PV module : MATLAB Function  TreatAsAtomicUnit=on
  Vpv array : powerlib/Measurements/Voltage Measurement  PhasorSimulation=off  OutputType=Complex  PSBequivalent=0
  + : PMIOPort  Tag=PMCPort  Port=1  Side=Right
  - : PMIOPort  Tag=PMCPort  Port=2  Side=Right
  Ipv : Outport
  Vpv : Outport  Port=2
  wires:
  Radiación/1 -> PV module/2(Radiacion)
  Temperatura/1 -> PV module/3(Temp)
  PV module/1(I) -> Controlled Current Source/1, Ipv/1
  Vpv array/1 -> PV module/1(V), Vpv/1
  connections:
  Controlled Current Source/LConn1 -- Diode/LConn1 -- -/RConn1 -- Vpv array/LConn2
  Controlled Current Source/RConn1 -- Diode/RConn1 -- +/RConn1 -- Vpv array/LConn1

== system ArregloSeisPorSeis/Array/PV panel2 ==
  Radiación : Inport
  Temperatura : Inport  Port=2
  Controlled Current Source : powerlib/Electrical Sources/Controlled Current Source  Initialize=on  Source_Type=AC  Amplitude=0  Phase=0  Frequency=0  Measurements=None
  Diode : powerlib/Power Electronics/Diode  Ron=0.001  Lon=0  Vf=0  IC=0  UseSnubber=off  Rs=500  Cs=250e-9  Measurements=off
  PV module : MATLAB Function  TreatAsAtomicUnit=on
  Vpv array : powerlib/Measurements/Voltage Measurement  PhasorSimulation=off  OutputType=Complex  PSBequivalent=0
  + : PMIOPort  Tag=PMCPort  Port=1  Side=Right
  - : PMIOPort  Tag=PMCPort  Port=2  Side=Right
  Ipv : Outport
  Vpv : Outport  Port=2
  wires:
  Radiación/1 -> PV module/2(Radiacion)
  Temperatura/1 -> PV module/3(Temp)
  PV module/1(I) -> Controlled Current Source/1, Ipv/1
  Vpv array/1 -> PV module/1(V), Vpv/1
  connections:
  Controlled Current Source/LConn1 -- Diode/LConn1 -- -/RConn1 -- Vpv array/LConn2
  Controlled Current Source/RConn1 -- Diode/RConn1 -- +/RConn1 -- Vpv array/LConn1

== system ArregloSeisPorSeis/Array/PV panel20 ==
  Radiación : Inport
  Temperatura : Inport  Port=2
  Controlled Current Source : powerlib/Electrical Sources/Controlled Current Source  Initialize=on  Source_Type=AC  Amplitude=0  Phase=0  Frequency=0  Measurements=None
  Diode : powerlib/Power Electronics/Diode  Ron=0.001  Lon=0  Vf=0  IC=0  UseSnubber=off  Rs=500  Cs=250e-9  Measurements=off
  PV module : MATLAB Function  TreatAsAtomicUnit=on
  Vpv array : powerlib/Measurements/Voltage Measurement  PhasorSimulation=off  OutputType=Complex  PSBequivalent=0
  + : PMIOPort  Tag=PMCPort  Port=1  Side=Right
  - : PMIOPort  Tag=PMCPort  Port=2  Side=Right
  Ipv : Outport
  Vpv : Outport  Port=2
  wires:
  Radiación/1 -> PV module/2(Radiacion)
  Temperatura/1 -> PV module/3(Temp)
  PV module/1(I) -> Controlled Current Source/1, Ipv/1
  Vpv array/1 -> PV module/1(V), Vpv/1
  connections:
  Controlled Current Source/LConn1 -- Diode/LConn1 -- -/RConn1 -- Vpv array/LConn2
  Controlled Current Source/RConn1 -- Diode/RConn1 -- +/RConn1 -- Vpv array/LConn1

== system ArregloSeisPorSeis/Array/PV panel21 ==
  Radiación : Inport
  Temperatura : Inport  Port=2
  Controlled Current Source : powerlib/Electrical Sources/Controlled Current Source  Initialize=on  Source_Type=AC  Amplitude=0  Phase=0  Frequency=0  Measurements=None
  Diode : powerlib/Power Electronics/Diode  Ron=0.001  Lon=0  Vf=0  IC=0  UseSnubber=off  Rs=500  Cs=250e-9  Measurements=off
  PV module : MATLAB Function  TreatAsAtomicUnit=on
  Vpv array : powerlib/Measurements/Voltage Measurement  PhasorSimulation=off  OutputType=Complex  PSBequivalent=0
  + : PMIOPort  Tag=PMCPort  Port=1  Side=Right
  - : PMIOPort  Tag=PMCPort  Port=2  Side=Right
  Ipv : Outport
  Vpv : Outport  Port=2
  wires:
  Radiación/1 -> PV module/2(Radiacion)
  Temperatura/1 -> PV module/3(Temp)
  PV module/1(I) -> Controlled Current Source/1, Ipv/1
  Vpv array/1 -> PV module/1(V), Vpv/1
  connections:
  Controlled Current Source/LConn1 -- Diode/LConn1 -- -/RConn1 -- Vpv array/LConn2
  Controlled Current Source/RConn1 -- Diode/RConn1 -- +/RConn1 -- Vpv array/LConn1

== system ArregloSeisPorSeis/Array/PV panel22 ==
  Radiación : Inport
  Temperatura : Inport  Port=2
  Controlled Current Source : powerlib/Electrical Sources/Controlled Current Source  Initialize=on  Source_Type=AC  Amplitude=0  Phase=0  Frequency=0  Measurements=None
  Diode : powerlib/Power Electronics/Diode  Ron=0.001  Lon=0  Vf=0  IC=0  UseSnubber=off  Rs=500  Cs=250e-9  Measurements=off
  PV module : MATLAB Function  TreatAsAtomicUnit=on
  Vpv array : powerlib/Measurements/Voltage Measurement  PhasorSimulation=off  OutputType=Complex  PSBequivalent=0
  + : PMIOPort  Tag=PMCPort  Port=1  Side=Right
  - : PMIOPort  Tag=PMCPort  Port=2  Side=Right
  Ipv : Outport
  Vpv : Outport  Port=2
  wires:
  Radiación/1 -> PV module/2(Radiacion)
  Temperatura/1 -> PV module/3(Temp)
  PV module/1(I) -> Controlled Current Source/1, Ipv/1
  Vpv array/1 -> PV module/1(V), Vpv/1
  connections:
  Controlled Current Source/LConn1 -- Diode/LConn1 -- -/RConn1 -- Vpv array/LConn2
  Controlled Current Source/RConn1 -- Diode/RConn1 -- +/RConn1 -- Vpv array/LConn1

== system ArregloSeisPorSeis/Array/PV panel23 ==
  Radiación : Inport
  Temperatura : Inport  Port=2
  Controlled Current Source : powerlib/Electrical Sources/Controlled Current Source  Initialize=on  Source_Type=AC  Amplitude=0  Phase=0  Frequency=0  Measurements=None
  Diode : powerlib/Power Electronics/Diode  Ron=0.001  Lon=0  Vf=0  IC=0  UseSnubber=off  Rs=500  Cs=250e-9  Measurements=off
  PV module : MATLAB Function  TreatAsAtomicUnit=on
  Vpv array : powerlib/Measurements/Voltage Measurement  PhasorSimulation=off  OutputType=Complex  PSBequivalent=0
  + : PMIOPort  Tag=PMCPort  Port=1  Side=Right
  - : PMIOPort  Tag=PMCPort  Port=2  Side=Right
  Ipv : Outport
  Vpv : Outport  Port=2
  wires:
  Radiación/1 -> PV module/2(Radiacion)
  Temperatura/1 -> PV module/3(Temp)
  PV module/1(I) -> Controlled Current Source/1, Ipv/1
  Vpv array/1 -> PV module/1(V), Vpv/1
  connections:
  Controlled Current Source/LConn1 -- Diode/LConn1 -- -/RConn1 -- Vpv array/LConn2
  Controlled Current Source/RConn1 -- Diode/RConn1 -- +/RConn1 -- Vpv array/LConn1

== system ArregloSeisPorSeis/Array/PV panel24 ==
  Radiación : Inport
  Temperatura : Inport  Port=2
  Controlled Current Source : powerlib/Electrical Sources/Controlled Current Source  Initialize=on  Source_Type=AC  Amplitude=0  Phase=0  Frequency=0  Measurements=None
  Diode : powerlib/Power Electronics/Diode  Ron=0.001  Lon=0  Vf=0  IC=0  UseSnubber=off  Rs=500  Cs=250e-9  Measurements=off
  PV module : MATLAB Function  TreatAsAtomicUnit=on
  Vpv array : powerlib/Measurements/Voltage Measurement  PhasorSimulation=off  OutputType=Complex  PSBequivalent=0
  + : PMIOPort  Tag=PMCPort  Port=1  Side=Right
  - : PMIOPort  Tag=PMCPort  Port=2  Side=Right
  Ipv : Outport
  Vpv : Outport  Port=2
  wires:
  Radiación/1 -> PV module/2(Radiacion)
  Temperatura/1 -> PV module/3(Temp)
  PV module/1(I) -> Controlled Current Source/1, Ipv/1
  Vpv array/1 -> PV module/1(V), Vpv/1
  connections:
  Controlled Current Source/LConn1 -- Diode/LConn1 -- -/RConn1 -- Vpv array/LConn2
  Controlled Current Source/RConn1 -- Diode/RConn1 -- +/RConn1 -- Vpv array/LConn1

== system ArregloSeisPorSeis/Array/PV panel25 ==
  Radiación : Inport
  Temperatura : Inport  Port=2
  Controlled Current Source : powerlib/Electrical Sources/Controlled Current Source  Initialize=on  Source_Type=AC  Amplitude=0  Phase=0  Frequency=0  Measurements=None
  Diode : powerlib/Power Electronics/Diode  Ron=0.001  Lon=0  Vf=0  IC=0  UseSnubber=off  Rs=500  Cs=250e-9  Measurements=off
  PV module : MATLAB Function  TreatAsAtomicUnit=on
  Vpv array : powerlib/Measurements/Voltage Measurement  PhasorSimulation=off  OutputType=Complex  PSBequivalent=0
  + : PMIOPort  Tag=PMCPort  Port=1  Side=Right
  - : PMIOPort  Tag=PMCPort  Port=2  Side=Right
  Ipv : Outport
  Vpv : Outport  Port=2
  wires:
  Radiación/1 -> PV module/2(Radiacion)
  Temperatura/1 -> PV module/3(Temp)
  PV module/1(I) -> Controlled Current Source/1, Ipv/1
  Vpv array/1 -> PV module/1(V), Vpv/1
  connections:
  Controlled Current Source/LConn1 -- Diode/LConn1 -- -/RConn1 -- Vpv array/LConn2
  Controlled Current Source/RConn1 -- Diode/RConn1 -- +/RConn1 -- Vpv array/LConn1

== system ArregloSeisPorSeis/Array/PV panel26 ==
  Radiación : Inport
  Temperatura : Inport  Port=2
  Controlled Current Source : powerlib/Electrical Sources/Controlled Current Source  Initialize=on  Source_Type=AC  Amplitude=0  Phase=0  Frequency=0  Measurements=None
  Diode : powerlib/Power Electronics/Diode  Ron=0.001  Lon=0  Vf=0  IC=0  UseSnubber=off  Rs=500  Cs=250e-9  Measurements=off
  PV module : MATLAB Function  TreatAsAtomicUnit=on
  Vpv array : powerlib/Measurements/Voltage Measurement  PhasorSimulation=off  OutputType=Complex  PSBequivalent=0
  + : PMIOPort  Tag=PMCPort  Port=1  Side=Right
  - : PMIOPort  Tag=PMCPort  Port=2  Side=Right
  Ipv : Outport
  Vpv : Outport  Port=2
  wires:
  Radiación/1 -> PV module/2(Radiacion)
  Temperatura/1 -> PV module/3(Temp)
  PV module/1(I) -> Controlled Current Source/1, Ipv/1
  Vpv array/1 -> PV module/1(V), Vpv/1
  connections:
  Controlled Current Source/LConn1 -- Diode/LConn1 -- -/RConn1 -- Vpv array/LConn2
  Controlled Current Source/RConn1 -- Diode/RConn1 -- +/RConn1 -- Vpv array/LConn1

== system ArregloSeisPorSeis/Array/PV panel27 ==
  Radiación : Inport
  Temperatura : Inport  Port=2
  Controlled Current Source : powerlib/Electrical Sources/Controlled Current Source  Initialize=on  Source_Type=AC  Amplitude=0  Phase=0  Frequency=0  Measurements=None
  Diode : powerlib/Power Electronics/Diode  Ron=0.001  Lon=0  Vf=0  IC=0  UseSnubber=off  Rs=500  Cs=250e-9  Measurements=off
  PV module : MATLAB Function  TreatAsAtomicUnit=on
  Vpv array : powerlib/Measurements/Voltage Measurement  PhasorSimulation=off  OutputType=Complex  PSBequivalent=0
  + : PMIOPort  Tag=PMCPort  Port=1  Side=Right
  - : PMIOPort  Tag=PMCPort  Port=2  Side=Right
  Ipv : Outport
  Vpv : Outport  Port=2
  wires:
  Radiación/1 -> PV module/2(Radiacion)
  Temperatura/1 -> PV module/3(Temp)
  PV module/1(I) -> Controlled Current Source/1, Ipv/1
  Vpv array/1 -> PV module/1(V), Vpv/1
  connections:
  Controlled Current Source/LConn1 -- Diode/LConn1 -- -/RConn1 -- Vpv array/LConn2
  Controlled Current Source/RConn1 -- Diode/RConn1 -- +/RConn1 -- Vpv array/LConn1

== system ArregloSeisPorSeis/Array/PV panel28 ==
  Radiación : Inport
  Temperatura : Inport  Port=2
  Controlled Current Source : powerlib/Electrical Sources/Controlled Current Source  Initialize=on  Source_Type=AC  Amplitude=0  Phase=0  Frequency=0  Measurements=None
  Diode : powerlib/Power Electronics/Diode  Ron=0.001  Lon=0  Vf=0  IC=0  UseSnubber=off  Rs=500  Cs=250e-9  Measurements=off
  PV module : MATLAB Function  TreatAsAtomicUnit=on
  Vpv array : powerlib/Measurements/Voltage Measurement  PhasorSimulation=off  OutputType=Complex  PSBequivalent=0
  + : PMIOPort  Tag=PMCPort  Port=1  Side=Right
  - : PMIOPort  Tag=PMCPort  Port=2  Side=Right
  Ipv : Outport
  Vpv : Outport  Port=2
  wires:
  Radiación/1 -> PV module/2(Radiacion)
  Temperatura/1 -> PV module/3(Temp)
  PV module/1(I) -> Controlled Current Source/1, Ipv/1
  Vpv array/1 -> PV module/1(V), Vpv/1
  connections:
  Controlled Current Source/LConn1 -- Diode/LConn1 -- -/RConn1 -- Vpv array/LConn2
  Controlled Current Source/RConn1 -- Diode/RConn1 -- +/RConn1 -- Vpv array/LConn1

== system ArregloSeisPorSeis/Array/PV panel29 ==
  Radiación : Inport
  Temperatura : Inport  Port=2
  Controlled Current Source : powerlib/Electrical Sources/Controlled Current Source  Initialize=on  Source_Type=AC  Amplitude=0  Phase=0  Frequency=0  Measurements=None
  Diode : powerlib/Power Electronics/Diode  Ron=0.001  Lon=0  Vf=0  IC=0  UseSnubber=off  Rs=500  Cs=250e-9  Measurements=off
  PV module : MATLAB Function  TreatAsAtomicUnit=on
  Vpv array : powerlib/Measurements/Voltage Measurement  PhasorSimulation=off  OutputType=Complex  PSBequivalent=0
  + : PMIOPort  Tag=PMCPort  Port=1  Side=Right
  - : PMIOPort  Tag=PMCPort  Port=2  Side=Right
  Ipv : Outport
  Vpv : Outport  Port=2
  wires:
  Radiación/1 -> PV module/2(Radiacion)
  Temperatura/1 -> PV module/3(Temp)
  PV module/1(I) -> Controlled Current Source/1, Ipv/1
  Vpv array/1 -> PV module/1(V), Vpv/1
  connections:
  Controlled Current Source/LConn1 -- Diode/LConn1 -- -/RConn1 -- Vpv array/LConn2
  Controlled Current Source/RConn1 -- Diode/RConn1 -- +/RConn1 -- Vpv array/LConn1

== system ArregloSeisPorSeis/Array/PV panel3 ==
  Radiación : Inport
  Temperatura : Inport  Port=2
  Controlled Current Source : powerlib/Electrical Sources/Controlled Current Source  Initialize=on  Source_Type=AC  Amplitude=0  Phase=0  Frequency=0  Measurements=None
  Diode : powerlib/Power Electronics/Diode  Ron=0.001  Lon=0  Vf=0  IC=0  UseSnubber=off  Rs=500  Cs=250e-9  Measurements=off
  PV module : MATLAB Function  TreatAsAtomicUnit=on
  Vpv array : powerlib/Measurements/Voltage Measurement  PhasorSimulation=off  OutputType=Complex  PSBequivalent=0
  + : PMIOPort  Tag=PMCPort  Port=1  Side=Right
  - : PMIOPort  Tag=PMCPort  Port=2  Side=Right
  Ipv : Outport
  Vpv : Outport  Port=2
  wires:
  Radiación/1 -> PV module/2(Radiacion)
  Temperatura/1 -> PV module/3(Temp)
  PV module/1(I) -> Controlled Current Source/1, Ipv/1
  Vpv array/1 -> PV module/1(V), Vpv/1
  connections:
  Controlled Current Source/LConn1 -- Diode/LConn1 -- -/RConn1 -- Vpv array/LConn2
  Controlled Current Source/RConn1 -- Diode/RConn1 -- +/RConn1 -- Vpv array/LConn1

== system ArregloSeisPorSeis/Array/PV panel30 ==
  Radiación : Inport
  Temperatura : Inport  Port=2
  Controlled Current Source : powerlib/Electrical Sources/Controlled Current Source  Initialize=on  Source_Type=AC  Amplitude=0  Phase=0  Frequency=0  Measurements=None
  Diode : powerlib/Power Electronics/Diode  Ron=0.001  Lon=0  Vf=0  IC=0  UseSnubber=off  Rs=500  Cs=250e-9  Measurements=off
  PV module : MATLAB Function  TreatAsAtomicUnit=on
  Vpv array : powerlib/Measurements/Voltage Measurement  PhasorSimulation=off  OutputType=Complex  PSBequivalent=0
  + : PMIOPort  Tag=PMCPort  Port=1  Side=Right
  - : PMIOPort  Tag=PMCPort  Port=2  Side=Right
  Ipv : Outport
  Vpv : Outport  Port=2
  wires:
  Radiación/1 -> PV module/2(Radiacion)
  Temperatura/1 -> PV module/3(Temp)
  PV module/1(I) -> Controlled Current Source/1, Ipv/1
  Vpv array/1 -> PV module/1(V), Vpv/1
  connections:
  Controlled Current Source/LConn1 -- Diode/LConn1 -- -/RConn1 -- Vpv array/LConn2
  Controlled Current Source/RConn1 -- Diode/RConn1 -- +/RConn1 -- Vpv array/LConn1

== system ArregloSeisPorSeis/Array/PV panel31 ==
  Radiación : Inport
  Temperatura : Inport  Port=2
  Controlled Current Source : powerlib/Electrical Sources/Controlled Current Source  Initialize=on  Source_Type=AC  Amplitude=0  Phase=0  Frequency=0  Measurements=None
  Diode : powerlib/Power Electronics/Diode  Ron=0.001  Lon=0  Vf=0  IC=0  UseSnubber=off  Rs=500  Cs=250e-9  Measurements=off
  PV module : MATLAB Function  TreatAsAtomicUnit=on
  Vpv array : powerlib/Measurements/Voltage Measurement  PhasorSimulation=off  OutputType=Complex  PSBequivalent=0
  + : PMIOPort  Tag=PMCPort  Port=1  Side=Right
  - : PMIOPort  Tag=PMCPort  Port=2  Side=Right
  Ipv : Outport
  Vpv : Outport  Port=2
  wires:
  Radiación/1 -> PV module/2(Radiacion)
  Temperatura/1 -> PV module/3(Temp)
  PV module/1(I) -> Controlled Current Source/1, Ipv/1
  Vpv array/1 -> PV module/1(V), Vpv/1
  connections:
  Controlled Current Source/LConn1 -- Diode/LConn1 -- -/RConn1 -- Vpv array/LConn2
  Controlled Current Source/RConn1 -- Diode/RConn1 -- +/RConn1 -- Vpv array/LConn1

== system ArregloSeisPorSeis/Array/PV panel32 ==
  Radiación : Inport
  Temperatura : Inport  Port=2
  Controlled Current Source : powerlib/Electrical Sources/Controlled Current Source  Initialize=on  Source_Type=AC  Amplitude=0  Phase=0  Frequency=0  Measurements=None
  Diode : powerlib/Power Electronics/Diode  Ron=0.001  Lon=0  Vf=0  IC=0  UseSnubber=off  Rs=500  Cs=250e-9  Measurements=off
  PV module : MATLAB Function  TreatAsAtomicUnit=on
  Vpv array : powerlib/Measurements/Voltage Measurement  PhasorSimulation=off  OutputType=Complex  PSBequivalent=0
  + : PMIOPort  Tag=PMCPort  Port=1  Side=Right
  - : PMIOPort  Tag=PMCPort  Port=2  Side=Right
  Ipv : Outport
  Vpv : Outport  Port=2
  wires:
  Radiación/1 -> PV module/2(Radiacion)
  Temperatura/1 -> PV module/3(Temp)
  PV module/1(I) -> Controlled Current Source/1, Ipv/1
  Vpv array/1 -> PV module/1(V), Vpv/1
  connections:
  Controlled Current Source/LConn1 -- Diode/LConn1 -- -/RConn1 -- Vpv array/LConn2
  Controlled Current Source/RConn1 -- Diode/RConn1 -- +/RConn1 -- Vpv array/LConn1

== system ArregloSeisPorSeis/Array/PV panel33 ==
  Radiación : Inport
  Temperatura : Inport  Port=2
  Controlled Current Source : powerlib/Electrical Sources/Controlled Current Source  Initialize=on  Source_Type=AC  Amplitude=0  Phase=0  Frequency=0  Measurements=None
  Diode : powerlib/Power Electronics/Diode  Ron=0.001  Lon=0  Vf=0  IC=0  UseSnubber=off  Rs=500  Cs=250e-9  Measurements=off
  PV module : MATLAB Function  TreatAsAtomicUnit=on
  Vpv array : powerlib/Measurements/Voltage Measurement  PhasorSimulation=off  OutputType=Complex  PSBequivalent=0
  + : PMIOPort  Tag=PMCPort  Port=1  Side=Right
  - : PMIOPort  Tag=PMCPort  Port=2  Side=Right
  Ipv : Outport
  Vpv : Outport  Port=2
  wires:
  Radiación/1 -> PV module/2(Radiacion)
  Temperatura/1 -> PV module/3(Temp)
  PV module/1(I) -> Controlled Current Source/1, Ipv/1
  Vpv array/1 -> PV module/1(V), Vpv/1
  connections:
  Controlled Current Source/LConn1 -- Diode/LConn1 -- -/RConn1 -- Vpv array/LConn2
  Controlled Current Source/RConn1 -- Diode/RConn1 -- +/RConn1 -- Vpv array/LConn1

== system ArregloSeisPorSeis/Array/PV panel34 ==
  Radiación : Inport
  Temperatura : Inport  Port=2
  Controlled Current Source : powerlib/Electrical Sources/Controlled Current Source  Initialize=on  Source_Type=AC  Amplitude=0  Phase=0  Frequency=0  Measurements=None
  Diode : powerlib/Power Electronics/Diode  Ron=0.001  Lon=0  Vf=0  IC=0  UseSnubber=off  Rs=500  Cs=250e-9  Measurements=off
  PV module : MATLAB Function  TreatAsAtomicUnit=on
  Vpv array : powerlib/Measurements/Voltage Measurement  PhasorSimulation=off  OutputType=Complex  PSBequivalent=0
  + : PMIOPort  Tag=PMCPort  Port=1  Side=Right
  - : PMIOPort  Tag=PMCPort  Port=2  Side=Right
  Ipv : Outport
  Vpv : Outport  Port=2
  wires:
  Radiación/1 -> PV module/2(Radiacion)
  Temperatura/1 -> PV module/3(Temp)
  PV module/1(I) -> Controlled Current Source/1, Ipv/1
  Vpv array/1 -> PV module/1(V), Vpv/1
  connections:
  Controlled Current Source/LConn1 -- Diode/LConn1 -- -/RConn1 -- Vpv array/LConn2
  Controlled Current Source/RConn1 -- Diode/RConn1 -- +/RConn1 -- Vpv array/LConn1
